simulink model "FlexPWM_simple_and_compl"  (Simulink 8.1)
settings: Solver=FixedStepDiscrete  StartTime=0.0  StopTime=50.0  FixedStep=1.0  RelTol=1e-3
undefined symbols (not defined in the file or in its folder): A10, A14, A15, B, B13, B7, C6, D, L3, PA12, PA13, PC10, PD4, R10
libraries: rappid_564xl_ec_toolbox x3
settings Model: Creator=evarshavskaya  LastModifiedBy=evarshavskaya
settings DataIOCC: ExternalInput=off  InitialState=off  SaveOutput=off  SignalLogging=off  SaveTime=off
settings OptimizationCC: InlineParams=on  OptimizeModelRefInitCode=on  LifeSpan=1
settings DebuggingCC: InheritedTsInSrcMsg=none  SingleTaskRateTransMsg=error  UnconnectedInputMsg=error  UnconnectedOutputMsg=error  UnconnectedLineMsg=error  UnknownTsInhSupMsg=error
settings HardwareCC: ProdLargestAtomicInteger=Long  ProdLargestAtomicFloat=Double  ProdIntDivRoundTo=Zero  ProdEndianess=BigEndian  ProdHWDeviceType=Freescale->32-bit PowerPC
settings RTWCC: SystemTargetFile=rappid564xl.tlc  MakeCommand=rappid_564xl_make_rtw  TemplateMakefile=rappid_564xl_default_tmf  PostCodeGenCommand=rappid_analyzegencode(buildInfo)  Description=RAppID Toolbox MPC564xL Code Generation Target (rappid)  ProcessScript=rappid564xl_make_rtw_hook
settings CodeAppCC: IgnoreCustomStorageClasses=off  CustomSymbolStrType=$N$R$M  InternalIdentifier=Classic
settings STFCustomTargetCC: CodeReplacementLibrary=ANSI_C  ModelReferenceCompliant=off  CombineOutputUpdateFcns=on  SuppressErrorStatus=on  ERTCustomFileBanners=on  SupportContinuousTime=off  SupportNonInlinedSFcns=off  MATLABClassNameForMDSCustomization=Simulink.SoftwareTarget.ERTCustomization  GRTInterface=off  SystemTargetFile=rappid564xl.tlc
settings ERTTargetCC: CodeReplacementLibrary=ANSI_C  MultiwordLength=2048  ModelReferenceCompliant=off  ParMdlRefBuildCompliant=off  CompOptLevelCompliant=off  ConcurrentExecutionCompliant=off  SuppressErrorStatus=on  ERTFirstTimeCompliant=off  ModelStepFunctionPrototypeControlCompliant=off  CPPClassGenCompliant=off  ExtModeMexFile=noextcomm  InlinedParameterPlacement=NonHierarchical  ERTCustomFileTemplate=example_file_process.tlc  ConvertIfToSwitch=off  SuppressUnreachableDefaultCases=off

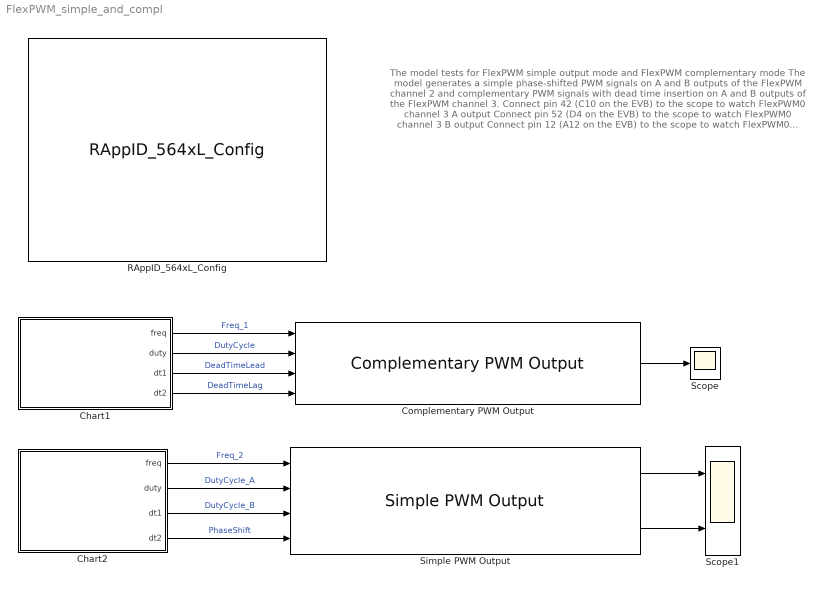
== system FlexPWM_simple_and_compl ==
  note: The model tests for FlexPWM simple output mode and FlexPWM complementary mode
      |
      | The model generates a simple phase-shifted PWM signals on A and B outputs of the FlexPWM channel 2
      | and complementary PWM signals with dead time insertion on A and B outputs of the FlexPWM channel 3.
      |
      | Connect pin 42 (C10 on the EVB) to the scope to watch FlexPWM0 channel 3 A output
      | Connect pin 52 (D4 on the EVB) to the scope to watch FlexPWM0 channel 3 B output
      | Connect pin 12 (A12 on the EVB) to the scope to watch FlexPWM0 channel 2 A output
      | Connect pin 13 (A13 on the EVB) to the scope to watch FlexPWM0 channel 2 B output
  Chart1 : Stateflow chart  TreatAsAtomicUnit=on
  Chart2 : Stateflow chart  TreatAsAtomicUnit=on
  Complementary PWM Output : rappid_564xl_ec_toolbox/MPC564xL/Motor Control Blocks/Complementary PWM Output  pwmModule=0  pwmMod=0  SubModule=3  subMod=3  InitFreq=1000  resolution=0.1 %  resValue=10  InitDuty=300  pwm45=off  pwm45en=0  InitDutyB=0  DeadTime=100  dt=IPBus clock cycles  deadtime_mks=0  debugSw=on  debug_mode=1  pin_A0=None  pin_B0=None  pin_A1=None  pin_B1=None  pin_A2=None  pin_B2=None  pin_A3="42  : PC10 : [ 111 ] : [ A15 ]"  pin_B3="52  : PD4  : [ 129 ] : [ B7 ]"  pin1_A0=None  pin1_B0=None  pin1_A1=None  pin1_B1=None  pin1_A2=None  pin1_B2=None  pin1_A3=None  pin1_B3=None  pcrNumA=42  pcrNumB=52  polA=off  polB=off  octrl=0  syncFrom0=off  masterSync=0  outVal0=off  outVal1=off  outVal2=on  outVal3=on  outVal4=on  outVal5=on  outTrig=12
  RAppID_564xL_Config : rappid_564xl_ec_toolbox/MPC564xL/RAppID_564xL_Config  SystemClock=120  XTAL=40  MC_clock_60=12  MC_clock_80=16  MC_clock_120=10  SWG_clock_60=20  SWG_clock_80=13.334  SWG_clock_120=20  Compiler=CodeWarrior  MemTarget=RAM  Part=MPC5643L  Package=144 LQFP  global_int_priority=10  base_tick_priority=14  sys_task_supress=off  exception_handlers=off  stored_mdl_name=FlexPWM_1  freemaster_interface=Oops  freemaster_rx_pin="LINFlex_0 Rx Pin 116 : \"PB[3]\""  freemaster_tx_pin="LINFlex_0 Tx Pin 114 : \"PB[2]\""  freemaster_interface_1=None  freemaster_enable=off  freemaster_rate=57600  freemaster_tx0_pin=18 : B[2] : 114 : A14  freemaster_rx0_pin=19 : B[3] : 116 : B13  freemaster_tx1_pin=57 : D[9] : 26 : L3  freemaster_rx1_pin=29 : B[13] : 60 : R10  freemaster_can_channel=1CH  freemater_can_speed=500K  freemaster_can_msgig=0x7AA  ccp_interface=None  ccp_enable=off  ccp_can_channel=CH1 (MB 0 - 1)  ccp_can_speed=500K  ccp_can_cro_id=256  ccp_can_dto_id=257  ccp_dev_id=RappID  ccp_dev_addr=0  ccp_odt=3  ccp_daq=3  pil_enable=off  pil_bam=on  comport=1  pil_rate=57600  bam_password_def=on  bam_password=0xFEEDFACECAFEBEEF  bam_sa_cs=off  bam_start_address=0x0  bam_code_size=0x7000  cons_dspi=on  cons_can=on  cons_adc=on  cons_pwm=on  cons_ctu=on  cons_swg=on  cons_eTimer=on  cons_fm=on
  Scope : Scope
      settings: TickLabels=on  TimeRange=50  YMin=0  YMax=1
  Scope1 : Scope  NumInputPorts=2
      settings: TickLabels=on  TimeRange=50  YMin=0~0  YMax=1~1
  Simple PWM Output : rappid_564xl_ec_toolbox/MPC564xL/Motor Control Blocks/Simple PWM Output  pwmModule=0  pwmMod=0  SubModule=2  subMod=2  InitFreq=2000  resolution=1 %  resValue=1  InitDutyA=60  InitDutyB=20  align=A - edge aligned B - phase shifted  PhaseShift_A=0  PhaseShift=30  Phase_A=0  Phase_B=30  centered=-1  DoubleS=off  doubleSw=off  debugSw=on  debug_mode=1  pin_A0=None  pin_B0=None  pin_X0=None  pin_A1=None  pin_B1=None  pin_X1=None  pin_A2="12  : PA12 : [ 122 ] : [ A10 ]"  pin_B2="13  : PA13 : [ 136 ] : [ C6 ]"  pin_X2=None  pin_A3=None  pin_B3=None  pin_X3=None  pin1_A0=None  pin1_B0=None  pin1_X0=None  pin1_A1=None  pin1_B1=None  pin1_X1=None  pin1_A2=None  pin1_B2=None  pin1_X2=None  pin1_A3=None  pin1_B3=None  pin1_X3=None  pcrNumA=12  pcrNumB=13  pcrNumX=255  polA=off  polB=off  polX=off  octrl=0  syncFrom0=off  masterSync=0  outVal0=off  outVal1=off  outVal2=on  outVal3=on  outVal4=on  outVal5=on  outTrig=60
  wires:
  Chart1/1(freq) -> Complementary PWM Output/1  "Freq_1"
  Chart1/2(duty) -> Complementary PWM Output/2  "DutyCycle"
  Chart1/3(dt1) -> Complementary PWM Output/3  "DeadTimeLead"
  Chart1/4(dt2) -> Complementary PWM Output/4  "DeadTimeLag"
  Complementary PWM Output/1 -> Scope/1
  Chart2/2(duty) -> Simple PWM Output/2  "DutyCycle_A"
  Chart2/3(dt1) -> Simple PWM Output/3  "DutyCycle_B"
  Chart2/4(dt2) -> Simple PWM Output/4  "PhaseShift"
  Chart2/1(freq) -> Simple PWM Output/1  "Freq_2"
  Simple PWM Output/1 -> Scope1/1
  Simple PWM Output/2 -> Scope1/2

== stateflow chart Chart2 ==
  settings: executeAtInitialization=1
  state A
    du:
    freq =2000;
    duty=60;
    dt1=20;
    dt2=30;
    cntr=cntr+1;
  state A1
    du:
    freq =2000;
    duty=40;
    dt1=30;
    dt2=60;
    cntr=cntr-1;
  (default) -> A : {cntr=0;}
  A1 -> A : [cntr < 2]
  A -> A1 : [cntr > 10]
  data: cntr local uint32 =0; freq output uint32; duty output uint32 [0..100]; dt1 output uint32; dt2 output uint32

== stateflow chart Chart1 ==
  settings: executeAtInitialization=1
  state A
    du:
    freq =1000;
    duty=700;
    dt1=100;
    dt2=100;
    cntr=cntr+1;
  state A1
    du:
    freq =1000;
    duty=300;
    dt1=200;
    dt2=200;
    cntr=cntr-1;
  (default) -> A : {cntr=0;}
  A1 -> A : [cntr < 2]
  A -> A1 : [cntr > 10]
  data: cntr local uint32 [0..1000] =0; freq output uint32 [0..10000]; duty output uint32 [0..1000]; dt1 output uint32 [0..4095]; dt2 output uint32 [0..4095]
